simulink model "Scenario_3_v2"  (R2020b)
settings: Solver=ode1be  StartTime=0.0  StopTime=0.5  FixedStep=Ts  MaxStep=Ts/10  MinStep=Ts/40  RelTol=1e-3
values from neighbouring files (symbols this model uses):
  c0 = c0_zeb    (= 6.57988e-09)    [Scenario_17_parameters_v2.m]    (also in Scenario_1_parameters_v2.m; Scenario_2_parameters_v2.m; Scenario_3_parameters_v2.m)
  c0_hawk = 6.37282e-09    [Scenario_17_parameters_v2.m]    (also in Scenario_1_parameters_v2.m; Scenario_2_parameters_v2.m; Scenario_3_parameters_v2.m)
  c1 = c1_zeb    (= 9.15905e-09)    [Scenario_17_parameters_v2.m]    (also in Scenario_1_parameters_v2.m; Scenario_2_parameters_v2.m; Scenario_3_parameters_v2.m)
  c1_hawk = 8.76156e-09    [Scenario_17_parameters_v2.m]    (also in Scenario_1_parameters_v2.m; Scenario_2_parameters_v2.m; Scenario_3_parameters_v2.m)
  fg = 50    [Scenario_17_parameters_v2.m]    (also in Scenario_1_parameters_v2.m; Scenario_2_parameters_v2.m; Scenario_3_parameters_v2.m)
  G10gen = 0.90    (= 0.9)    [Scenario_3_parameters_v2.m]
  G12gen = 0.85    [Scenario_3_parameters_v2.m]
  G1gen = 0.4692    [Scenario_17_parameters_v2.m]    (also in Scenario_1_parameters_v2.m = 0.1; Scenario_2_parameters_v2.m = 0.298581; Scenario_3_parameters_v2.m = 0.65)
  G2gen = 0.80    (= 0.8)    [Scenario_1_parameters_v2.m]    (also in Scenario_2_parameters_v2.m = 0.7; Scenario_3_parameters_v2.m = 0.4)
  G3gen = 0.85    [Scenario_1_parameters_v2.m]    (also in Scenario_2_parameters_v2.m = 0.9; Scenario_3_parameters_v2.m = 0.6)
  G4gen = 0.65    [Scenario_3_parameters_v2.m]
  G5gen = 0.75    [Scenario_17_parameters_v2.m]    (also in Scenario_1_parameters_v2.m = 0.8; Scenario_2_parameters_v2.m = 0.8; Scenario_3_parameters_v2.m = 0.705)
  G6gen = 0.90    (= 0.9)    [Scenario_17_parameters_v2.m]    (also in Scenario_1_parameters_v2.m; Scenario_2_parameters_v2.m = 0.81797; Scenario_3_parameters_v2.m = 0.45)
  G7gen = 0.20    (= 0.2)    [Scenario_17_parameters_v2.m]    (also in Scenario_1_parameters_v2.m = 0.5227; Scenario_2_parameters_v2.m = 0.5098; Scenario_3_parameters_v2.m = 0.4)
  G8gen = 0.58    [Scenario_17_parameters_v2.m]    (also in Scenario_3_parameters_v2.m = 0.65)
  G9gen = 0.8833    [Scenario_17_parameters_v2.m]    (also in Scenario_3_parameters_v2.m = 0.9)
  Iovc = 1.2    [Scenario_17_parameters_v2.m]    (also in Scenario_1_parameters_v2.m; Scenario_2_parameters_v2.m; Scenario_3_parameters_v2.m)
  l0 = l0_zeb    (= 0.00368)    [Scenario_17_parameters_v2.m]    (also in Scenario_1_parameters_v2.m; Scenario_2_parameters_v2.m; Scenario_3_parameters_v2.m)
  l0_hawk = 0.00373    [Scenario_17_parameters_v2.m]    (also in Scenario_1_parameters_v2.m; Scenario_2_parameters_v2.m; Scenario_3_parameters_v2.m)
  l1 = l1_zeb    (= 0.00128)    [Scenario_17_parameters_v2.m]    (also in Scenario_1_parameters_v2.m; Scenario_2_parameters_v2.m; Scenario_3_parameters_v2.m)
  L10dem = 0.04    [Scenario_3_parameters_v2.m]
  L12dem = 0.01    [Scenario_17_parameters_v2.m]    (also in Scenario_3_parameters_v2.m = 0.02)
  L13dem = 0.01    [Scenario_3_parameters_v2.m]
  l1_hawk = 0.00133    [Scenario_17_parameters_v2.m]    (also in Scenario_1_parameters_v2.m; Scenario_2_parameters_v2.m; Scenario_3_parameters_v2.m)
  L1dem = 0.25    [Scenario_17_parameters_v2.m]    (also in Scenario_3_parameters_v2.m = 0.1)
  L3dem = 0.30    (= 0.3)    [Scenario_17_parameters_v2.m]    (also in Scenario_1_parameters_v2.m = 0.1; Scenario_2_parameters_v2.m = 0.1; Scenario_3_parameters_v2.m = 0.2)
  L5dem = 0.25    [Scenario_17_parameters_v2.m]    (also in Scenario_1_parameters_v2.m = 0.35; Scenario_2_parameters_v2.m = 0.35; Scenario_3_parameters_v2.m = 0.1)
  L6dem = 0.15    [Scenario_1_parameters_v2.m]    (also in Scenario_2_parameters_v2.m; Scenario_3_parameters_v2.m = 0.1)
  L7dem = 0.10    (= 0.1)    [Scenario_1_parameters_v2.m]    (also in Scenario_2_parameters_v2.m; Scenario_3_parameters_v2.m = 0.2)
  L9dem = 0.15    [Scenario_17_parameters_v2.m]    (also in Scenario_3_parameters_v2.m = 0.1)
  Pr = Sr*PF    (= 1600500000)    [Scenario_17_parameters_v2.m]    (also in Scenario_1_parameters_v2.m = 1472500000; Scenario_2_parameters_v2.m = 1805000000; Scenario_3_parameters_v2.m = 12740000000)
  Qr = sqrt(Sr^2 - Pr^2)    [Scenario_17_parameters_v2.m]    (also in Scenario_1_parameters_v2.m; Scenario_2_parameters_v2.m; Scenario_3_parameters_v2.m)
  r0 = r0_zeb    (= 0.39362)    [Scenario_17_parameters_v2.m]    (also in Scenario_1_parameters_v2.m; Scenario_2_parameters_v2.m; Scenario_3_parameters_v2.m)
  r0_hawk = 0.44587    [Scenario_17_parameters_v2.m]    (also in Scenario_1_parameters_v2.m; Scenario_2_parameters_v2.m; Scenario_3_parameters_v2.m)
  r1 = r1_zeb    (= 0.06862)    [Scenario_17_parameters_v2.m]    (also in Scenario_1_parameters_v2.m; Scenario_2_parameters_v2.m; Scenario_3_parameters_v2.m)
  r1_hawk = 0.12087    [Scenario_17_parameters_v2.m]    (also in Scenario_1_parameters_v2.m; Scenario_2_parameters_v2.m; Scenario_3_parameters_v2.m)
  Rtpu = Xtpu/40    (= 0.0025)    [Scenario_17_parameters_v2.m]    (also in Scenario_1_parameters_v2.m = 0.00375; Scenario_2_parameters_v2.m = 0.00375; Scenario_3_parameters_v2.m)
  S10non = 500e6    (= 500000000)    [Scenario_3_parameters_v2.m]
  S12non = 250e6    (= 250000000)    [Scenario_3_parameters_v2.m]
  S1non = 700e6    (= 700000000)    [Scenario_17_parameters_v2.m]    (also in Scenario_1_parameters_v2.m = 400000000; Scenario_2_parameters_v2.m = 400000000; Scenario_3_parameters_v2.m = 1000000000)
  S2non = 300e6    (= 300000000)    [Scenario_1_parameters_v2.m]    (also in Scenario_2_parameters_v2.m; Scenario_3_parameters_v2.m = 3000000000)
  S3non = 200e6    (= 200000000)    [Scenario_1_parameters_v2.m]    (also in Scenario_2_parameters_v2.m; Scenario_3_parameters_v2.m = 1000000000)
  S4non = 2000e6    (= 2000000000)    [Scenario_3_parameters_v2.m]
  S5non = 400e6    (= 400000000)    [Scenario_17_parameters_v2.m]    (also in Scenario_1_parameters_v2.m = 500000000; Scenario_2_parameters_v2.m = 500000000; Scenario_3_parameters_v2.m = 2000000000)
  S6non = 150e6    (= 150000000)    [Scenario_17_parameters_v2.m]    (also in Scenario_1_parameters_v2.m = 400000000; Scenario_2_parameters_v2.m = 400000000; Scenario_3_parameters_v2.m = 3000000000)
  S7non = 1500e6    (= 1500000000)    [Scenario_17_parameters_v2.m]    (also in Scenario_1_parameters_v2.m = 200000000; Scenario_2_parameters_v2.m = 200000000; Scenario_3_parameters_v2.m = 4000000000)
  S8non = 600e6    (= 600000000)    [Scenario_17_parameters_v2.m]    (also in Scenario_3_parameters_v2.m = 2000000000)
  S9non = 200e6    (= 200000000)    [Scenario_17_parameters_v2.m]    (also in Scenario_3_parameters_v2.m = 1500000000)
  tonvsc = 0    [Scenario_17_parameters_v2.m]    (also in Scenario_1_parameters_v2.m; Scenario_2_parameters_v2.m; Scenario_3_parameters_v2.m = 0.0001)
  Ts = 50e-6    (= 5e-05)    [Scenario_17_parameters_v2.m]    (also in Scenario_1_parameters_v2.m = 0.0002; Scenario_2_parameters_v2.m = 2e-05; Scenario_3_parameters_v2.m = 0.0001)
  Vhv = 220e3    (= 220000)    [Scenario_17_parameters_v2.m]    (also in Scenario_1_parameters_v2.m; Scenario_2_parameters_v2.m; Scenario_3_parameters_v2.m)
  Vmv = 22e3    (= 22000)    [Scenario_17_parameters_v2.m]    (also in Scenario_1_parameters_v2.m; Scenario_2_parameters_v2.m; Scenario_3_parameters_v2.m)
  w_pll = 2*pi*80    (= 502.654824574)    [Scenario_17_parameters_v2.m]    (also in Scenario_1_parameters_v2.m; Scenario_2_parameters_v2.m; Scenario_3_parameters_v2.m)
  wc1 = wsw1/10    (= 848.230016469)    [Scenario_17_parameters_v2.m]    (also in Scenario_1_parameters_v2.m; Scenario_2_parameters_v2.m; Scenario_3_parameters_v2.m)
  wdc1 = wc1/10    (= 84.8230016469)    [Scenario_17_parameters_v2.m]    (also in Scenario_1_parameters_v2.m; Scenario_2_parameters_v2.m; Scenario_3_parameters_v2.m)
  wpq1 = wc1/10    (= 84.8230016469)    [Scenario_17_parameters_v2.m]    (also in Scenario_1_parameters_v2.m; Scenario_2_parameters_v2.m; Scenario_3_parameters_v2.m)
  wsw1 = ksw1*2*pi*fg    (= 8482.30016469)    [Scenario_17_parameters_v2.m]    (also in Scenario_1_parameters_v2.m; Scenario_2_parameters_v2.m; Scenario_3_parameters_v2.m)
  Xtpu = 0.10    (= 0.1)    [Scenario_17_parameters_v2.m]    (also in Scenario_1_parameters_v2.m = 0.15; Scenario_2_parameters_v2.m = 0.15; Scenario_3_parameters_v2.m)
undefined symbols (not defined in the file or in its folder): D11, Delta
libraries: powerlib x428, simulink_extras x272, powerlib_meascontrol x194, pid_lib x105, simulink x60, eeTransforms x54, spsFirstOrderFilterLib x36, eePwmGeneratorTwoLevel x9
(part 39 of 40)

== system Scenario_3_v2/G4/VSC v2/VSC Control/Control loops/Phasor PQ 1st/Outer-loop/Power calculation ==
  note: AC power calculation using symmetrical components in dq axis
  note: Pavgp = 3/2*(vqp*iqp + vdp*idp) and Qavgp = 3/2*(vqp*idp-vdp*iqp)
  note: P = Pavg + Pc2*cos(2wt) + Ps2*sin(2wt) ---> Pavg = Pavgp + Pavgn
  note: Q = Qavg + Qc2*cos(2wt) + Qs2*sin(2wt) ---> Qavg = Qavgp + Qavgn
  note: Pavgn = 3/2*(vqn*iqn + vdn*idn) and Qavgn = 3/2*(vqn*idn-vdn*iqn)
  vq+ : Inport
  vd+ : Inport  Port=2
  iq+ : Inport  Port=3
  id+ : Inport  Port=4
  vq- : Inport  Port=5
  vd- : Inport  Port=6
  iq- : Inport  Port=7
  id- : Inport  Port=8
  Gain : Gain  Gain=3/2
  Gain1 : Gain  Gain=3/2
  Gain2 : Gain  Gain=-1
  Gain3 : Gain  Gain=-1
  Gain4 : Gain  Gain=negseq_en
  Mux{,1..3} (4 alike) : Mux  Inputs=2
  Product{,1..3} (4 alike) : Product
  Sum1 : Sum
  Sum2 : Sum
  Sum8 : Sum
  PQ : Outport
  wires:
  Sum8/1 -> Gain/1
  Gain2/1 -> Mux2/2
  Mux2/1 -> Product2/2
  Product2/1 -> Sum8/2
  Mux/1 -> Product/2
  Product/1 -> Sum8/1
  iq+/1 -> [iqp]
  [iqp] -> Gain2/1, Mux/1
  id+/1 -> [idp]
  [idp] -> Mux2/1, Mux/2
  vq+/1 -> [vqp]
  [vqp] -> Product/1
  vd+/1 -> [vdp]
  [vdp] -> Product2/1
  Gain/1 -> Sum1/1
  Sum1/1 -> PQ/1
  Gain3/1 -> Mux3/2
  Mux1/1 -> Product1/2
  Product3/1 -> Sum2/2
  Product1/1 -> Sum2/1
  [vdn] -> Product3/1
  Mux3/1 -> Product3/2
  [vqn] -> Product1/1
  Sum2/1 -> Gain1/1
  [iqn] -> Gain3/1, Mux1/1
  [idn] -> Mux3/1, Mux1/2
  vq-/1 -> [vqn]
  vd-/1 -> [vdn]
  iq-/1 -> [iqn]
  id-/1 -> [idn]
  Gain1/1 -> Gain4/1
  Gain4/1 -> Sum1/2

== system Scenario_3_v2/G4/VSC v2/VSC Control/Control loops/SW, EMT AVG, Phasor Quasi-EMT/Outer-loop/Power calculation ==
  note: AC power calculation using symmetrical components in dq axis
  note: Pavgp = 3/2*(vqp*iqp + vdp*idp) and Qavgp = 3/2*(vqp*idp-vdp*iqp)
  note: P = Pavg + Pc2*cos(2wt) + Ps2*sin(2wt) ---> Pavg = Pavgp + Pavgn
  note: Q = Qavg + Qc2*cos(2wt) + Qs2*sin(2wt) ---> Qavg = Qavgp + Qavgn
  note: Pavgn = 3/2*(vqn*iqn + vdn*idn) and Qavgn = 3/2*(vqn*idn-vdn*iqn)
  vq+ : Inport
  vd+ : Inport  Port=2
  iq+ : Inport  Port=3
  id+ : Inport  Port=4
  vq- : Inport  Port=5
  vd- : Inport  Port=6
  iq- : Inport  Port=7
  id- : Inport  Port=8
  Gain : Gain  Gain=3/2
  Gain1 : Gain  Gain=3/2
  Gain2 : Gain  Gain=-1
  Gain3 : Gain  Gain=-1
  Gain4 : Gain  Gain=negseq_en
  Mux{,1..3} (4 alike) : Mux  Inputs=2
  Product{,1..3} (4 alike) : Product
  Sum1 : Sum
  Sum2 : Sum
  Sum8 : Sum
  PQ : Outport
  wires:
  Sum8/1 -> Gain/1
  Gain2/1 -> Mux2/2
  Mux2/1 -> Product2/2
  Product2/1 -> Sum8/2
  Mux/1 -> Product/2
  Product/1 -> Sum8/1
  iq+/1 -> [iqp]
  [iqp] -> Gain2/1, Mux/1
  id+/1 -> [idp]
  [idp] -> Mux2/1, Mux/2
  vq+/1 -> [vqp]
  [vqp] -> Product/1
  vd+/1 -> [vdp]
  [vdp] -> Product2/1
  Gain/1 -> Sum1/1
  Sum1/1 -> PQ/1
  Gain3/1 -> Mux3/2
  Mux1/1 -> Product1/2
  Product3/1 -> Sum2/2
  Product1/1 -> Sum2/1
  [vdn] -> Product3/1
  Mux3/1 -> Product3/2
  [vqn] -> Product1/1
  Sum2/1 -> Gain1/1
  [iqn] -> Gain3/1, Mux1/1
  [idn] -> Mux3/1, Mux1/2
  vq-/1 -> [vqn]
  vd-/1 -> [vdn]
  iq-/1 -> [iqn]
  id-/1 -> [idn]
  Gain1/1 -> Gain4/1
  Gain4/1 -> Sum1/2

== system Scenario_3_v2/G4/VSC v2/VSC Control/Control loops/SW, EMT AVG, Phasor Quasi-EMT/Outer-loop/Subsystem2 ==
  note: Hold initial variable value for a given time
  In1 : Inport
  Constant : Constant  Value=x0
  Constant1 : Constant
  Integrator : Integrator
  Switch : Switch  Threshold=Td
  Out1 : Outport
  wires:
  Integrator/1 -> Switch/2
  In1/1 -> Switch/1
  Switch/1 -> Out1/1
  Constant/1 -> Switch/3
  Constant1/1 -> Integrator/1

== system Scenario_3_v2/G4/VSC v2/VSC Control/Control loops/SW, EMT AVG, Phasor Quasi-EMT/Outer-loop/Subsystem3 ==
  note: Hold initial variable value for a given time
  In1 : Inport
  Constant : Constant  Value=x0
  Constant1 : Constant
  Integrator : Integrator
  Switch : Switch  Threshold=Td
  Out1 : Outport
  wires:
  Integrator/1 -> Switch/2
  In1/1 -> Switch/1
  Switch/1 -> Out1/1
  Constant/1 -> Switch/3
  Constant1/1 -> Integrator/1

== system Scenario_3_v2/G4/VSC v2/VSC Control/Measurements/EMT/PLL aligned with positive-sequence/Phase-sequence separation ==
  note: Phase-sequence separation based on
      | Delayed Signal Cancellation (DSC) method
  abc : Inport
  Theta : Inport  Port=2
  Complex to Real-Imag1 : ComplexToRealImag
  Complex to Real-Imag2 : ComplexToRealImag
  Complex to Real-Imag3 : ComplexToRealImag
  Constant : Constant  Value=negseq_en
  Demux3 : Demux  Outputs=3
  Exp2 : Math  OutputSignalType=complex  SaturateOnIntegerOverflow=on
  Exp3 : Math  OutputSignalType=complex  SaturateOnIntegerOverflow=on
  Gain1 : Gain  Gain=1/2
  Gain4 : Gain  Gain=-1i
  Gain5 : Gain  Gain=1i
  Gain6 : Gain  Gain=1/2
  Gain7 : Gain  Gain=1i
  NOT : Logic  Operator=NOT  IconShape=distinctive  AllPortsSameDT=off  OutDataTypeStr=boolean
  Product3 : Product
  Product4 : Product
  Real-Imag to Complex : RealImagToComplex
  Real-Imag to Complex1 : RealImagToComplex
  Sum1 : Sum  Inputs=|++
  Sum2 : Sum  Inputs=-+|
  Switch : Switch  Criteria=u2 ~= 0
  Terminator3 : Terminator
  Transport Delay2 : TransportDelay  DelayTime=1/4*(1/fg)  BufferSize=1024*4
  Transport Delay3 : TransportDelay  DelayTime=1/4*(1/fg)  BufferSize=1024*4
  abc to Alpha-Beta-Zero : powerlib_meascontrol/Transformations/abc to Alpha-Beta-Zero
  q+ : Outport
  d+ : Outport  Port=2
  q- : Outport  Port=3
  d- : Outport  Port=4
  wires:
  NOT/1 -> Switch/2
  Constant/1 -> NOT/1
  Switch/1 -> Product3/1
  Gain6/1 -> Switch/3
  Sum2/1 -> Gain1/1
  Transport Delay2/1 -> Real-Imag to Complex1/1
  Demux3/1 -> Real-Imag to Complex/1
  Complex to Real-Imag1/2 -> Transport Delay3/1
  Gain1/1 -> Product4/2
  Real-Imag to Complex/1 -> Complex to Real-Imag1/1, Sum2/2, Sum1/1, Switch/1
  Complex to Real-Imag3/1 -> d-/1
  Real-Imag to Complex1/1 -> Gain5/1
  Complex to Real-Imag1/1 -> Transport Delay2/1
  Transport Delay3/1 -> Real-Imag to Complex1/2
  Demux3/2 -> Real-Imag to Complex/2
  Product3/1 -> Complex to Real-Imag2/1
  Product4/1 -> Complex to Real-Imag3/1
  abc to Alpha-Beta-Zero/1 -> Demux3/1
  abc/1 -> abc to Alpha-Beta-Zero/1
  Exp3/1 -> Product4/1
  Complex to Real-Imag3/2 -> q-/1
  Complex to Real-Imag2/2 -> q+/1
  Demux3/3 -> Terminator3/1
  Sum1/1 -> Gain6/1
  Gain5/1 -> Sum2/1, Sum1/2
  Exp2/1 -> Product3/2
  Gain4/1 -> Exp2/1
  Theta/1 -> Gain4/1, Gain7/1
  Gain7/1 -> Exp3/1
  Complex to Real-Imag2/1 -> d+/1

== system Scenario_3_v2/G4/VSC v2/VSC Control/Measurements/EMT/PLL aligned with positive-sequence/Subsystem ==
  note: PI controller with reset port and initial conditions restored after reset or after maximum/minimum values are reached
  in : Inport
  Reset : Inport  Port=2
  Compare To Constant2 : simulink/Logic and Bit Operations/Compare To Constant  relop=~=  const=0  OutDataTypeStr=boolean
  Constant2 : Constant  Value=2*pi*fg
  Gain : Gain  Gain=kp_pll
  Gain1 : Gain  Gain=kp_pll/tau_pll
  Integrator Limited : Integrator  ExternalReset=level  InitialCondition=2*pi*fg  UpperSaturationLimit=10.1*2*pi*fg  LowerSaturationLimit=0.09*2*pi*fg  ShowSaturationPort=on
  Memory1 : Memory
  NOT : Logic  Operator=NOT  IconShape=distinctive  AllPortsSameDT=off  OutDataTypeStr=boolean
  OR2 : Logic  Operator=OR  IconShape=distinctive  AllPortsSameDT=off  OutDataTypeStr=boolean
  Product : Product
  Sum : Sum
  Switch1 : Switch
  w : Outport
  wires:
  Switch1/1 -> w/1
  Product/1 -> Gain1/1, Gain/1
  Gain1/1 -> Integrator Limited/1
  Integrator Limited/2 -> Compare To Constant2/1, Switch1/2
  Compare To Constant2/1 -> Memory1/1
  OR2/1 -> Integrator Limited/2, NOT/1
  Constant2/1 -> Switch1/3
  Memory1/1 -> OR2/1
  Reset/1 -> OR2/2
  Gain/1 -> Sum/1
  Integrator Limited/1 -> Sum/2
  Sum/1 -> Switch1/1
  in/1 -> Product/1
  NOT/1 -> Product/2

== system Scenario_3_v2/G6/VSC v2/VSC Control/Control loops/Phasor I 1st/Outer-loop/Power calculation ==
  note: AC power calculation using symmetrical components in dq axis
  note: Pavgp = 3/2*(vqp*iqp + vdp*idp) and Qavgp = 3/2*(vqp*idp-vdp*iqp)
  note: P = Pavg + Pc2*cos(2wt) + Ps2*sin(2wt) ---> Pavg = Pavgp + Pavgn
  note: Q = Qavg + Qc2*cos(2wt) + Qs2*sin(2wt) ---> Qavg = Qavgp + Qavgn
  note: Pavgn = 3/2*(vqn*iqn + vdn*idn) and Qavgn = 3/2*(vqn*idn-vdn*iqn)
  vq+ : Inport
  vd+ : Inport  Port=2
  iq+ : Inport  Port=3
  id+ : Inport  Port=4
  vq- : Inport  Port=5
  vd- : Inport  Port=6
  iq- : Inport  Port=7
  id- : Inport  Port=8
  Gain : Gain  Gain=3/2
  Gain1 : Gain  Gain=3/2
  Gain2 : Gain  Gain=-1
  Gain3 : Gain  Gain=-1
  Gain4 : Gain  Gain=negseq_en
  Mux{,1..3} (4 alike) : Mux  Inputs=2
  Product{,1..3} (4 alike) : Product
  Sum1 : Sum
  Sum2 : Sum
  Sum8 : Sum
  PQ : Outport
  wires:
  Sum8/1 -> Gain/1
  Gain2/1 -> Mux2/2
  Mux2/1 -> Product2/2
  Product2/1 -> Sum8/2
  Mux/1 -> Product/2
  Product/1 -> Sum8/1
  iq+/1 -> [iqp]
  [iqp] -> Gain2/1, Mux/1
  id+/1 -> [idp]
  [idp] -> Mux2/1, Mux/2
  vq+/1 -> [vqp]
  [vqp] -> Product/1
  vd+/1 -> [vdp]
  [vdp] -> Product2/1
  Gain/1 -> Sum1/1
  Sum1/1 -> PQ/1
  Gain3/1 -> Mux3/2
  Mux1/1 -> Product1/2
  Product3/1 -> Sum2/2
  Product1/1 -> Sum2/1
  [vdn] -> Product3/1
  Mux3/1 -> Product3/2
  [vqn] -> Product1/1
  Sum2/1 -> Gain1/1
  [iqn] -> Gain3/1, Mux1/1
  [idn] -> Mux3/1, Mux1/2
  vq-/1 -> [vqn]
  vd-/1 -> [vdn]
  iq-/1 -> [iqn]
  id-/1 -> [idn]
  Gain1/1 -> Gain4/1
  Gain4/1 -> Sum1/2

== system Scenario_3_v2/G6/VSC v2/VSC Control/Control loops/Phasor I ref/Outer-loop/Power calculation ==
  note: AC power calculation using symmetrical components in dq axis
  note: Pavgp = 3/2*(vqp*iqp + vdp*idp) and Qavgp = 3/2*(vqp*idp-vdp*iqp)
  note: P = Pavg + Pc2*cos(2wt) + Ps2*sin(2wt) ---> Pavg = Pavgp + Pavgn
  note: Q = Qavg + Qc2*cos(2wt) + Qs2*sin(2wt) ---> Qavg = Qavgp + Qavgn
  note: Pavgn = 3/2*(vqn*iqn + vdn*idn) and Qavgn = 3/2*(vqn*idn-vdn*iqn)
  vq+ : Inport
  vd+ : Inport  Port=2
  iq+ : Inport  Port=3
  id+ : Inport  Port=4
  vq- : Inport  Port=5
  vd- : Inport  Port=6
  iq- : Inport  Port=7
  id- : Inport  Port=8
  Gain : Gain  Gain=3/2
  Gain1 : Gain  Gain=3/2
  Gain2 : Gain  Gain=-1
  Gain3 : Gain  Gain=-1
  Gain4 : Gain  Gain=negseq_en
  Mux{,1..3} (4 alike) : Mux  Inputs=2
  Product{,1..3} (4 alike) : Product
  Sum1 : Sum
  Sum2 : Sum
  Sum8 : Sum
  PQ : Outport
  wires:
  Sum8/1 -> Gain/1
  Gain2/1 -> Mux2/2
  Mux2/1 -> Product2/2
  Product2/1 -> Sum8/2
  Mux/1 -> Product/2
  Product/1 -> Sum8/1
  iq+/1 -> [iqp]
  [iqp] -> Gain2/1, Mux/1
  id+/1 -> [idp]
  [idp] -> Mux2/1, Mux/2
  vq+/1 -> [vqp]
  [vqp] -> Product/1
  vd+/1 -> [vdp]
  [vdp] -> Product2/1
  Gain/1 -> Sum1/1
  Sum1/1 -> PQ/1
  Gain3/1 -> Mux3/2
  Mux1/1 -> Product1/2
  Product3/1 -> Sum2/2
  Product1/1 -> Sum2/1
  [vdn] -> Product3/1
  Mux3/1 -> Product3/2
  [vqn] -> Product1/1
  Sum2/1 -> Gain1/1
  [iqn] -> Gain3/1, Mux1/1
  [idn] -> Mux3/1, Mux1/2
  vq-/1 -> [vqn]
  vd-/1 -> [vdn]
  iq-/1 -> [iqn]
  id-/1 -> [idn]
  Gain1/1 -> Gain4/1
  Gain4/1 -> Sum1/2

== system Scenario_3_v2/G6/VSC v2/VSC Control/Control loops/Phasor PQ 1st/Outer-loop/Power calculation ==
  note: AC power calculation using symmetrical components in dq axis
  note: Pavgp = 3/2*(vqp*iqp + vdp*idp) and Qavgp = 3/2*(vqp*idp-vdp*iqp)
  note: P = Pavg + Pc2*cos(2wt) + Ps2*sin(2wt) ---> Pavg = Pavgp + Pavgn
  note: Q = Qavg + Qc2*cos(2wt) + Qs2*sin(2wt) ---> Qavg = Qavgp + Qavgn
  note: Pavgn = 3/2*(vqn*iqn + vdn*idn) and Qavgn = 3/2*(vqn*idn-vdn*iqn)
  vq+ : Inport
  vd+ : Inport  Port=2
  iq+ : Inport  Port=3
  id+ : Inport  Port=4
  vq- : Inport  Port=5
  vd- : Inport  Port=6
  iq- : Inport  Port=7
  id- : Inport  Port=8
  Gain : Gain  Gain=3/2
  Gain1 : Gain  Gain=3/2
  Gain2 : Gain  Gain=-1
  Gain3 : Gain  Gain=-1
  Gain4 : Gain  Gain=negseq_en
  Mux{,1..3} (4 alike) : Mux  Inputs=2
  Product{,1..3} (4 alike) : Product
  Sum1 : Sum
  Sum2 : Sum
  Sum8 : Sum
  PQ : Outport
  wires:
  Sum8/1 -> Gain/1
  Gain2/1 -> Mux2/2
  Mux2/1 -> Product2/2
  Product2/1 -> Sum8/2
  Mux/1 -> Product/2
  Product/1 -> Sum8/1
  iq+/1 -> [iqp]
  [iqp] -> Gain2/1, Mux/1
  id+/1 -> [idp]
  [idp] -> Mux2/1, Mux/2
  vq+/1 -> [vqp]
  [vqp] -> Product/1
  vd+/1 -> [vdp]
  [vdp] -> Product2/1
  Gain/1 -> Sum1/1
  Sum1/1 -> PQ/1
  Gain3/1 -> Mux3/2
  Mux1/1 -> Product1/2
  Product3/1 -> Sum2/2
  Product1/1 -> Sum2/1
  [vdn] -> Product3/1
  Mux3/1 -> Product3/2
  [vqn] -> Product1/1
  Sum2/1 -> Gain1/1
  [iqn] -> Gain3/1, Mux1/1
  [idn] -> Mux3/1, Mux1/2
  vq-/1 -> [vqn]
  vd-/1 -> [vdn]
  iq-/1 -> [iqn]
  id-/1 -> [idn]
  Gain1/1 -> Gain4/1
  Gain4/1 -> Sum1/2

== system Scenario_3_v2/G6/VSC v2/VSC Control/Control loops/SW, EMT AVG, Phasor Quasi-EMT/Outer-loop/Power calculation ==
  note: AC power calculation using symmetrical components in dq axis
  note: Pavgp = 3/2*(vqp*iqp + vdp*idp) and Qavgp = 3/2*(vqp*idp-vdp*iqp)
  note: P = Pavg + Pc2*cos(2wt) + Ps2*sin(2wt) ---> Pavg = Pavgp + Pavgn
  note: Q = Qavg + Qc2*cos(2wt) + Qs2*sin(2wt) ---> Qavg = Qavgp + Qavgn
  note: Pavgn = 3/2*(vqn*iqn + vdn*idn) and Qavgn = 3/2*(vqn*idn-vdn*iqn)
  vq+ : Inport
  vd+ : Inport  Port=2
  iq+ : Inport  Port=3
  id+ : Inport  Port=4
  vq- : Inport  Port=5
  vd- : Inport  Port=6
  iq- : Inport  Port=7
  id- : Inport  Port=8
  Gain : Gain  Gain=3/2
  Gain1 : Gain  Gain=3/2
  Gain2 : Gain  Gain=-1
  Gain3 : Gain  Gain=-1
  Gain4 : Gain  Gain=negseq_en
  Mux{,1..3} (4 alike) : Mux  Inputs=2
  Product{,1..3} (4 alike) : Product
  Sum1 : Sum
  Sum2 : Sum
  Sum8 : Sum
  PQ : Outport
  wires:
  Sum8/1 -> Gain/1
  Gain2/1 -> Mux2/2
  Mux2/1 -> Product2/2
  Product2/1 -> Sum8/2
  Mux/1 -> Product/2
  Product/1 -> Sum8/1
  iq+/1 -> [iqp]
  [iqp] -> Gain2/1, Mux/1
  id+/1 -> [idp]
  [idp] -> Mux2/1, Mux/2
  vq+/1 -> [vqp]
  [vqp] -> Product/1
  vd+/1 -> [vdp]
  [vdp] -> Product2/1
  Gain/1 -> Sum1/1
  Sum1/1 -> PQ/1
  Gain3/1 -> Mux3/2
  Mux1/1 -> Product1/2
  Product3/1 -> Sum2/2
  Product1/1 -> Sum2/1
  [vdn] -> Product3/1
  Mux3/1 -> Product3/2
  [vqn] -> Product1/1
  Sum2/1 -> Gain1/1
  [iqn] -> Gain3/1, Mux1/1
  [idn] -> Mux3/1, Mux1/2
  vq-/1 -> [vqn]
  vd-/1 -> [vdn]
  iq-/1 -> [iqn]
  id-/1 -> [idn]
  Gain1/1 -> Gain4/1
  Gain4/1 -> Sum1/2

== system Scenario_3_v2/G6/VSC v2/VSC Control/Control loops/SW, EMT AVG, Phasor Quasi-EMT/Outer-loop/Subsystem2 ==
  note: Hold initial variable value for a given time
  In1 : Inport
  Constant : Constant  Value=x0
  Constant1 : Constant
  Integrator : Integrator
  Switch : Switch  Threshold=Td
  Out1 : Outport
  wires:
  Integrator/1 -> Switch/2
  In1/1 -> Switch/1
  Switch/1 -> Out1/1
  Constant/1 -> Switch/3
  Constant1/1 -> Integrator/1

== system Scenario_3_v2/G6/VSC v2/VSC Control/Control loops/SW, EMT AVG, Phasor Quasi-EMT/Outer-loop/Subsystem3 ==
  note: Hold initial variable value for a given time
  In1 : Inport
  Constant : Constant  Value=x0
  Constant1 : Constant
  Integrator : Integrator
  Switch : Switch  Threshold=Td
  Out1 : Outport
  wires:
  Integrator/1 -> Switch/2
  In1/1 -> Switch/1
  Switch/1 -> Out1/1
  Constant/1 -> Switch/3
  Constant1/1 -> Integrator/1

== system Scenario_3_v2/G6/VSC v2/VSC Control/Measurements/EMT/PLL aligned with positive-sequence/Phase-sequence separation ==
  note: Phase-sequence separation based on
      | Delayed Signal Cancellation (DSC) method
  abc : Inport
  Theta : Inport  Port=2
  Complex to Real-Imag1 : ComplexToRealImag
  Complex to Real-Imag2 : ComplexToRealImag
  Complex to Real-Imag3 : ComplexToRealImag
  Constant : Constant  Value=negseq_en
  Demux3 : Demux  Outputs=3
  Exp2 : Math  OutputSignalType=complex  SaturateOnIntegerOverflow=on
  Exp3 : Math  OutputSignalType=complex  SaturateOnIntegerOverflow=on
  Gain1 : Gain  Gain=1/2
  Gain4 : Gain  Gain=-1i
  Gain5 : Gain  Gain=1i
  Gain6 : Gain  Gain=1/2
  Gain7 : Gain  Gain=1i
  NOT : Logic  Operator=NOT  IconShape=distinctive  AllPortsSameDT=off  OutDataTypeStr=boolean
  Product3 : Product
  Product4 : Product
  Real-Imag to Complex : RealImagToComplex
  Real-Imag to Complex1 : RealImagToComplex
  Sum1 : Sum  Inputs=|++
  Sum2 : Sum  Inputs=-+|
  Switch : Switch  Criteria=u2 ~= 0
  Terminator3 : Terminator
  Transport Delay2 : TransportDelay  DelayTime=1/4*(1/fg)  BufferSize=1024*4
  Transport Delay3 : TransportDelay  DelayTime=1/4*(1/fg)  BufferSize=1024*4
  abc to Alpha-Beta-Zero : powerlib_meascontrol/Transformations/abc to Alpha-Beta-Zero
  q+ : Outport
  d+ : Outport  Port=2
  q- : Outport  Port=3
  d- : Outport  Port=4
  wires:
  NOT/1 -> Switch/2
  Constant/1 -> NOT/1
  Switch/1 -> Product3/1
  Gain6/1 -> Switch/3
  Sum2/1 -> Gain1/1
  Transport Delay2/1 -> Real-Imag to Complex1/1
  Demux3/1 -> Real-Imag to Complex/1
  Complex to Real-Imag1/2 -> Transport Delay3/1
  Gain1/1 -> Product4/2
  Real-Imag to Complex/1 -> Complex to Real-Imag1/1, Sum2/2, Sum1/1, Switch/1
  Complex to Real-Imag3/1 -> d-/1
  Real-Imag to Complex1/1 -> Gain5/1
  Complex to Real-Imag1/1 -> Transport Delay2/1
  Transport Delay3/1 -> Real-Imag to Complex1/2
  Demux3/2 -> Real-Imag to Complex/2
  Product3/1 -> Complex to Real-Imag2/1
  Product4/1 -> Complex to Real-Imag3/1
  abc to Alpha-Beta-Zero/1 -> Demux3/1
  abc/1 -> abc to Alpha-Beta-Zero/1
  Exp3/1 -> Product4/1
  Complex to Real-Imag3/2 -> q-/1
  Complex to Real-Imag2/2 -> q+/1
  Demux3/3 -> Terminator3/1
  Sum1/1 -> Gain6/1
  Gain5/1 -> Sum2/1, Sum1/2
  Exp2/1 -> Product3/2
  Gain4/1 -> Exp2/1
  Theta/1 -> Gain4/1, Gain7/1
  Gain7/1 -> Exp3/1
  Complex to Real-Imag2/1 -> d+/1

== system Scenario_3_v2/G6/VSC v2/VSC Control/Measurements/EMT/PLL aligned with positive-sequence/Subsystem ==
  note: PI controller with reset port and initial conditions restored after reset or after maximum/minimum values are reached
  in : Inport
  Reset : Inport  Port=2
  Compare To Constant2 : simulink/Logic and Bit Operations/Compare To Constant  relop=~=  const=0  OutDataTypeStr=boolean
  Constant2 : Constant  Value=2*pi*fg
  Gain : Gain  Gain=kp_pll
  Gain1 : Gain  Gain=kp_pll/tau_pll
  Integrator Limited : Integrator  ExternalReset=level  InitialCondition=2*pi*fg  UpperSaturationLimit=10.1*2*pi*fg  LowerSaturationLimit=0.09*2*pi*fg  ShowSaturationPort=on
  Memory1 : Memory
  NOT : Logic  Operator=NOT  IconShape=distinctive  AllPortsSameDT=off  OutDataTypeStr=boolean
  OR2 : Logic  Operator=OR  IconShape=distinctive  AllPortsSameDT=off  OutDataTypeStr=boolean
  Product : Product
  Sum : Sum
  Switch1 : Switch
  w : Outport
  wires:
  Switch1/1 -> w/1
  Product/1 -> Gain1/1, Gain/1
  Gain1/1 -> Integrator Limited/1
  Integrator Limited/2 -> Compare To Constant2/1, Switch1/2
  Compare To Constant2/1 -> Memory1/1
  OR2/1 -> Integrator Limited/2, NOT/1
  Constant2/1 -> Switch1/3
  Memory1/1 -> OR2/1
  Reset/1 -> OR2/2
  Gain/1 -> Sum/1
  Integrator Limited/1 -> Sum/2
  Sum/1 -> Switch1/1
  in/1 -> Product/1
  NOT/1 -> Product/2

== system Scenario_3_v2/G7/VSC v2/VSC Control/Control loops/Phasor I 1st/Outer-loop/Power calculation ==
  note: AC power calculation using symmetrical components in dq axis
  note: Pavgp = 3/2*(vqp*iqp + vdp*idp) and Qavgp = 3/2*(vqp*idp-vdp*iqp)
  note: P = Pavg + Pc2*cos(2wt) + Ps2*sin(2wt) ---> Pavg = Pavgp + Pavgn
  note: Q = Qavg + Qc2*cos(2wt) + Qs2*sin(2wt) ---> Qavg = Qavgp + Qavgn
  note: Pavgn = 3/2*(vqn*iqn + vdn*idn) and Qavgn = 3/2*(vqn*idn-vdn*iqn)
  vq+ : Inport
  vd+ : Inport  Port=2
  iq+ : Inport  Port=3
  id+ : Inport  Port=4
  vq- : Inport  Port=5
  vd- : Inport  Port=6
  iq- : Inport  Port=7
  id- : Inport  Port=8
  Gain : Gain  Gain=3/2
  Gain1 : Gain  Gain=3/2
  Gain2 : Gain  Gain=-1
  Gain3 : Gain  Gain=-1
  Gain4 : Gain  Gain=negseq_en
  Mux{,1..3} (4 alike) : Mux  Inputs=2
  Product{,1..3} (4 alike) : Product
  Sum1 : Sum
  Sum2 : Sum
  Sum8 : Sum
  PQ : Outport
  wires:
  Sum8/1 -> Gain/1
  Gain2/1 -> Mux2/2
  Mux2/1 -> Product2/2
  Product2/1 -> Sum8/2
  Mux/1 -> Product/2
  Product/1 -> Sum8/1
  iq+/1 -> [iqp]
  [iqp] -> Gain2/1, Mux/1
  id+/1 -> [idp]
  [idp] -> Mux2/1, Mux/2
  vq+/1 -> [vqp]
  [vqp] -> Product/1
  vd+/1 -> [vdp]
  [vdp] -> Product2/1
  Gain/1 -> Sum1/1
  Sum1/1 -> PQ/1
  Gain3/1 -> Mux3/2
  Mux1/1 -> Product1/2
  Product3/1 -> Sum2/2
  Product1/1 -> Sum2/1
  [vdn] -> Product3/1
  Mux3/1 -> Product3/2
  [vqn] -> Product1/1
  Sum2/1 -> Gain1/1
  [iqn] -> Gain3/1, Mux1/1
  [idn] -> Mux3/1, Mux1/2
  vq-/1 -> [vqn]
  vd-/1 -> [vdn]
  iq-/1 -> [iqn]
  id-/1 -> [idn]
  Gain1/1 -> Gain4/1
  Gain4/1 -> Sum1/2

== system Scenario_3_v2/G7/VSC v2/VSC Control/Control loops/Phasor I ref/Outer-loop/Power calculation ==
  note: AC power calculation using symmetrical components in dq axis
  note: Pavgp = 3/2*(vqp*iqp + vdp*idp) and Qavgp = 3/2*(vqp*idp-vdp*iqp)
  note: P = Pavg + Pc2*cos(2wt) + Ps2*sin(2wt) ---> Pavg = Pavgp + Pavgn
  note: Q = Qavg + Qc2*cos(2wt) + Qs2*sin(2wt) ---> Qavg = Qavgp + Qavgn
  note: Pavgn = 3/2*(vqn*iqn + vdn*idn) and Qavgn = 3/2*(vqn*idn-vdn*iqn)
  vq+ : Inport
  vd+ : Inport  Port=2
  iq+ : Inport  Port=3
  id+ : Inport  Port=4
  vq- : Inport  Port=5
  vd- : Inport  Port=6
  iq- : Inport  Port=7
  id- : Inport  Port=8
  Gain : Gain  Gain=3/2
  Gain1 : Gain  Gain=3/2
  Gain2 : Gain  Gain=-1
  Gain3 : Gain  Gain=-1
  Gain4 : Gain  Gain=negseq_en
  Mux{,1..3} (4 alike) : Mux  Inputs=2
  Product{,1..3} (4 alike) : Product
  Sum1 : Sum
  Sum2 : Sum
  Sum8 : Sum
  PQ : Outport
  wires:
  Sum8/1 -> Gain/1
  Gain2/1 -> Mux2/2
  Mux2/1 -> Product2/2
  Product2/1 -> Sum8/2
  Mux/1 -> Product/2
  Product/1 -> Sum8/1
  iq+/1 -> [iqp]
  [iqp] -> Gain2/1, Mux/1
  id+/1 -> [idp]
  [idp] -> Mux2/1, Mux/2
  vq+/1 -> [vqp]
  [vqp] -> Product/1
  vd+/1 -> [vdp]
  [vdp] -> Product2/1
  Gain/1 -> Sum1/1
  Sum1/1 -> PQ/1
  Gain3/1 -> Mux3/2
  Mux1/1 -> Product1/2
  Product3/1 -> Sum2/2
  Product1/1 -> Sum2/1
  [vdn] -> Product3/1
  Mux3/1 -> Product3/2
  [vqn] -> Product1/1
  Sum2/1 -> Gain1/1
  [iqn] -> Gain3/1, Mux1/1
  [idn] -> Mux3/1, Mux1/2
  vq-/1 -> [vqn]
  vd-/1 -> [vdn]
  iq-/1 -> [iqn]
  id-/1 -> [idn]
  Gain1/1 -> Gain4/1
  Gain4/1 -> Sum1/2

== system Scenario_3_v2/G7/VSC v2/VSC Control/Control loops/Phasor PQ 1st/Outer-loop/Power calculation ==
  note: AC power calculation using symmetrical components in dq axis
  note: Pavgp = 3/2*(vqp*iqp + vdp*idp) and Qavgp = 3/2*(vqp*idp-vdp*iqp)
  note: P = Pavg + Pc2*cos(2wt) + Ps2*sin(2wt) ---> Pavg = Pavgp + Pavgn
  note: Q = Qavg + Qc2*cos(2wt) + Qs2*sin(2wt) ---> Qavg = Qavgp + Qavgn
  note: Pavgn = 3/2*(vqn*iqn + vdn*idn) and Qavgn = 3/2*(vqn*idn-vdn*iqn)
  vq+ : Inport
  vd+ : Inport  Port=2
  iq+ : Inport  Port=3
  id+ : Inport  Port=4
  vq- : Inport  Port=5
  vd- : Inport  Port=6
  iq- : Inport  Port=7
  id- : Inport  Port=8
  Gain : Gain  Gain=3/2
  Gain1 : Gain  Gain=3/2
  Gain2 : Gain  Gain=-1
  Gain3 : Gain  Gain=-1
  Gain4 : Gain  Gain=negseq_en
  Mux{,1..3} (4 alike) : Mux  Inputs=2
  Product{,1..3} (4 alike) : Product
  Sum1 : Sum
  Sum2 : Sum
  Sum8 : Sum
  PQ : Outport
  wires:
  Sum8/1 -> Gain/1
  Gain2/1 -> Mux2/2
  Mux2/1 -> Product2/2
  Product2/1 -> Sum8/2
  Mux/1 -> Product/2
  Product/1 -> Sum8/1
  iq+/1 -> [iqp]
  [iqp] -> Gain2/1, Mux/1
  id+/1 -> [idp]
  [idp] -> Mux2/1, Mux/2
  vq+/1 -> [vqp]
  [vqp] -> Product/1
  vd+/1 -> [vdp]
  [vdp] -> Product2/1
  Gain/1 -> Sum1/1
  Sum1/1 -> PQ/1
  Gain3/1 -> Mux3/2
  Mux1/1 -> Product1/2
  Product3/1 -> Sum2/2
  Product1/1 -> Sum2/1
  [vdn] -> Product3/1
  Mux3/1 -> Product3/2
  [vqn] -> Product1/1
  Sum2/1 -> Gain1/1
  [iqn] -> Gain3/1, Mux1/1
  [idn] -> Mux3/1, Mux1/2
  vq-/1 -> [vqn]
  vd-/1 -> [vdn]
  iq-/1 -> [iqn]
  id-/1 -> [idn]
  Gain1/1 -> Gain4/1
  Gain4/1 -> Sum1/2

== system Scenario_3_v2/G7/VSC v2/VSC Control/Control loops/SW, EMT AVG, Phasor Quasi-EMT/Outer-loop/Power calculation ==
  note: AC power calculation using symmetrical components in dq axis
  note: Pavgp = 3/2*(vqp*iqp + vdp*idp) and Qavgp = 3/2*(vqp*idp-vdp*iqp)
  note: P = Pavg + Pc2*cos(2wt) + Ps2*sin(2wt) ---> Pavg = Pavgp + Pavgn
  note: Q = Qavg + Qc2*cos(2wt) + Qs2*sin(2wt) ---> Qavg = Qavgp + Qavgn
  note: Pavgn = 3/2*(vqn*iqn + vdn*idn) and Qavgn = 3/2*(vqn*idn-vdn*iqn)
  vq+ : Inport
  vd+ : Inport  Port=2
  iq+ : Inport  Port=3
  id+ : Inport  Port=4
  vq- : Inport  Port=5
  vd- : Inport  Port=6
  iq- : Inport  Port=7
  id- : Inport  Port=8
  Gain : Gain  Gain=3/2
  Gain1 : Gain  Gain=3/2
  Gain2 : Gain  Gain=-1
  Gain3 : Gain  Gain=-1
  Gain4 : Gain  Gain=negseq_en
  Mux{,1..3} (4 alike) : Mux  Inputs=2
  Product{,1..3} (4 alike) : Product
  Sum1 : Sum
  Sum2 : Sum
  Sum8 : Sum
  PQ : Outport
  wires:
  Sum8/1 -> Gain/1
  Gain2/1 -> Mux2/2
  Mux2/1 -> Product2/2
  Product2/1 -> Sum8/2
  Mux/1 -> Product/2
  Product/1 -> Sum8/1
  iq+/1 -> [iqp]
  [iqp] -> Gain2/1, Mux/1
  id+/1 -> [idp]
  [idp] -> Mux2/1, Mux/2
  vq+/1 -> [vqp]
  [vqp] -> Product/1
  vd+/1 -> [vdp]
  [vdp] -> Product2/1
  Gain/1 -> Sum1/1
  Sum1/1 -> PQ/1
  Gain3/1 -> Mux3/2
  Mux1/1 -> Product1/2
  Product3/1 -> Sum2/2
  Product1/1 -> Sum2/1
  [vdn] -> Product3/1
  Mux3/1 -> Product3/2
  [vqn] -> Product1/1
  Sum2/1 -> Gain1/1
  [iqn] -> Gain3/1, Mux1/1
  [idn] -> Mux3/1, Mux1/2
  vq-/1 -> [vqn]
  vd-/1 -> [vdn]
  iq-/1 -> [iqn]
  id-/1 -> [idn]
  Gain1/1 -> Gain4/1
  Gain4/1 -> Sum1/2

== system Scenario_3_v2/G7/VSC v2/VSC Control/Control loops/SW, EMT AVG, Phasor Quasi-EMT/Outer-loop/Subsystem2 ==
  note: Hold initial variable value for a given time
  In1 : Inport
  Constant : Constant  Value=x0
  Constant1 : Constant
  Integrator : Integrator
  Switch : Switch  Threshold=Td
  Out1 : Outport
  wires:
  Integrator/1 -> Switch/2
  In1/1 -> Switch/1
  Switch/1 -> Out1/1
  Constant/1 -> Switch/3
  Constant1/1 -> Integrator/1

== system Scenario_3_v2/G7/VSC v2/VSC Control/Control loops/SW, EMT AVG, Phasor Quasi-EMT/Outer-loop/Subsystem3 ==
  note: Hold initial variable value for a given time
  In1 : Inport
  Constant : Constant  Value=x0
  Constant1 : Constant
  Integrator : Integrator
  Switch : Switch  Threshold=Td
  Out1 : Outport
  wires:
  Integrator/1 -> Switch/2
  In1/1 -> Switch/1
  Switch/1 -> Out1/1
  Constant/1 -> Switch/3
  Constant1/1 -> Integrator/1

== system Scenario_3_v2/G7/VSC v2/VSC Control/Measurements/EMT/PLL aligned with positive-sequence/Phase-sequence separation ==
  note: Phase-sequence separation based on
      | Delayed Signal Cancellation (DSC) method
  abc : Inport
  Theta : Inport  Port=2
  Complex to Real-Imag1 : ComplexToRealImag
  Complex to Real-Imag2 : ComplexToRealImag
  Complex to Real-Imag3 : ComplexToRealImag
  Constant : Constant  Value=negseq_en
  Demux3 : Demux  Outputs=3
  Exp2 : Math  OutputSignalType=complex  SaturateOnIntegerOverflow=on
  Exp3 : Math  OutputSignalType=complex  SaturateOnIntegerOverflow=on
  Gain1 : Gain  Gain=1/2
  Gain4 : Gain  Gain=-1i
  Gain5 : Gain  Gain=1i
  Gain6 : Gain  Gain=1/2
  Gain7 : Gain  Gain=1i
  NOT : Logic  Operator=NOT  IconShape=distinctive  AllPortsSameDT=off  OutDataTypeStr=boolean
  Product3 : Product
  Product4 : Product
  Real-Imag to Complex : RealImagToComplex
  Real-Imag to Complex1 : RealImagToComplex
  Sum1 : Sum  Inputs=|++
  Sum2 : Sum  Inputs=-+|
  Switch : Switch  Criteria=u2 ~= 0
  Terminator3 : Terminator
  Transport Delay2 : TransportDelay  DelayTime=1/4*(1/fg)  BufferSize=1024*4
  Transport Delay3 : TransportDelay  DelayTime=1/4*(1/fg)  BufferSize=1024*4
  abc to Alpha-Beta-Zero : powerlib_meascontrol/Transformations/abc to Alpha-Beta-Zero
  q+ : Outport
  d+ : Outport  Port=2
  q- : Outport  Port=3
  d- : Outport  Port=4
  wires:
  NOT/1 -> Switch/2
  Constant/1 -> NOT/1
  Switch/1 -> Product3/1
  Gain6/1 -> Switch/3
  Sum2/1 -> Gain1/1
  Transport Delay2/1 -> Real-Imag to Complex1/1
  Demux3/1 -> Real-Imag to Complex/1
  Complex to Real-Imag1/2 -> Transport Delay3/1
  Gain1/1 -> Product4/2
  Real-Imag to Complex/1 -> Complex to Real-Imag1/1, Sum2/2, Sum1/1, Switch/1
  Complex to Real-Imag3/1 -> d-/1
  Real-Imag to Complex1/1 -> Gain5/1
  Complex to Real-Imag1/1 -> Transport Delay2/1
  Transport Delay3/1 -> Real-Imag to Complex1/2
  Demux3/2 -> Real-Imag to Complex/2
  Product3/1 -> Complex to Real-Imag2/1
  Product4/1 -> Complex to Real-Imag3/1
  abc to Alpha-Beta-Zero/1 -> Demux3/1
  abc/1 -> abc to Alpha-Beta-Zero/1
  Exp3/1 -> Product4/1
  Complex to Real-Imag3/2 -> q-/1
  Complex to Real-Imag2/2 -> q+/1
  Demux3/3 -> Terminator3/1
  Sum1/1 -> Gain6/1
  Gain5/1 -> Sum2/1, Sum1/2
  Exp2/1 -> Product3/2
  Gain4/1 -> Exp2/1
  Theta/1 -> Gain4/1, Gain7/1
  Gain7/1 -> Exp3/1
  Complex to Real-Imag2/1 -> d+/1

== system Scenario_3_v2/G7/VSC v2/VSC Control/Measurements/EMT/PLL aligned with positive-sequence/Subsystem ==
  note: PI controller with reset port and initial conditions restored after reset or after maximum/minimum values are reached
  in : Inport
  Reset : Inport  Port=2
  Compare To Constant2 : simulink/Logic and Bit Operations/Compare To Constant  relop=~=  const=0  OutDataTypeStr=boolean
  Constant2 : Constant  Value=2*pi*fg
  Gain : Gain  Gain=kp_pll
  Gain1 : Gain  Gain=kp_pll/tau_pll
  Integrator Limited : Integrator  ExternalReset=level  InitialCondition=2*pi*fg  UpperSaturationLimit=10.1*2*pi*fg  LowerSaturationLimit=0.09*2*pi*fg  ShowSaturationPort=on
  Memory1 : Memory
  NOT : Logic  Operator=NOT  IconShape=distinctive  AllPortsSameDT=off  OutDataTypeStr=boolean
  OR2 : Logic  Operator=OR  IconShape=distinctive  AllPortsSameDT=off  OutDataTypeStr=boolean
  Product : Product
  Sum : Sum
  Switch1 : Switch
  w : Outport
  wires:
  Switch1/1 -> w/1
  Product/1 -> Gain1/1, Gain/1
  Gain1/1 -> Integrator Limited/1
  Integrator Limited/2 -> Compare To Constant2/1, Switch1/2
  Compare To Constant2/1 -> Memory1/1
  OR2/1 -> Integrator Limited/2, NOT/1
  Constant2/1 -> Switch1/3
  Memory1/1 -> OR2/1
  Reset/1 -> OR2/2
  Gain/1 -> Sum/1
  Integrator Limited/1 -> Sum/2
  Sum/1 -> Switch1/1
  in/1 -> Product/1
  NOT/1 -> Product/2

== system Scenario_3_v2/G9/VSC v2/VSC Control/Control loops/Phasor I 1st/Outer-loop/Power calculation ==
  note: AC power calculation using symmetrical components in dq axis
  note: Pavgp = 3/2*(vqp*iqp + vdp*idp) and Qavgp = 3/2*(vqp*idp-vdp*iqp)
  note: P = Pavg + Pc2*cos(2wt) + Ps2*sin(2wt) ---> Pavg = Pavgp + Pavgn
  note: Q = Qavg + Qc2*cos(2wt) + Qs2*sin(2wt) ---> Qavg = Qavgp + Qavgn
  note: Pavgn = 3/2*(vqn*iqn + vdn*idn) and Qavgn = 3/2*(vqn*idn-vdn*iqn)
  vq+ : Inport
  vd+ : Inport  Port=2
  iq+ : Inport  Port=3
  id+ : Inport  Port=4
  vq- : Inport  Port=5
  vd- : Inport  Port=6
  iq- : Inport  Port=7
  id- : Inport  Port=8
  Gain : Gain  Gain=3/2
  Gain1 : Gain  Gain=3/2
  Gain2 : Gain  Gain=-1
  Gain3 : Gain  Gain=-1
  Gain4 : Gain  Gain=negseq_en
  Mux{,1..3} (4 alike) : Mux  Inputs=2
  Product{,1..3} (4 alike) : Product
  Sum1 : Sum
  Sum2 : Sum
  Sum8 : Sum
  PQ : Outport
  wires:
  Sum8/1 -> Gain/1
  Gain2/1 -> Mux2/2
  Mux2/1 -> Product2/2
  Product2/1 -> Sum8/2
  Mux/1 -> Product/2
  Product/1 -> Sum8/1
  iq+/1 -> [iqp]
  [iqp] -> Gain2/1, Mux/1
  id+/1 -> [idp]
  [idp] -> Mux2/1, Mux/2
  vq+/1 -> [vqp]
  [vqp] -> Product/1
  vd+/1 -> [vdp]
  [vdp] -> Product2/1
  Gain/1 -> Sum1/1
  Sum1/1 -> PQ/1
  Gain3/1 -> Mux3/2
  Mux1/1 -> Product1/2
  Product3/1 -> Sum2/2
  Product1/1 -> Sum2/1
  [vdn] -> Product3/1
  Mux3/1 -> Product3/2
  [vqn] -> Product1/1
  Sum2/1 -> Gain1/1
  [iqn] -> Gain3/1, Mux1/1
  [idn] -> Mux3/1, Mux1/2
  vq-/1 -> [vqn]
  vd-/1 -> [vdn]
  iq-/1 -> [iqn]
  id-/1 -> [idn]
  Gain1/1 -> Gain4/1
  Gain4/1 -> Sum1/2

== system Scenario_3_v2/G9/VSC v2/VSC Control/Control loops/Phasor I ref/Outer-loop/Power calculation ==
  note: AC power calculation using symmetrical components in dq axis
  note: Pavgp = 3/2*(vqp*iqp + vdp*idp) and Qavgp = 3/2*(vqp*idp-vdp*iqp)
  note: P = Pavg + Pc2*cos(2wt) + Ps2*sin(2wt) ---> Pavg = Pavgp + Pavgn
  note: Q = Qavg + Qc2*cos(2wt) + Qs2*sin(2wt) ---> Qavg = Qavgp + Qavgn
  note: Pavgn = 3/2*(vqn*iqn + vdn*idn) and Qavgn = 3/2*(vqn*idn-vdn*iqn)
  vq+ : Inport
  vd+ : Inport  Port=2
  iq+ : Inport  Port=3
  id+ : Inport  Port=4
  vq- : Inport  Port=5
  vd- : Inport  Port=6
  iq- : Inport  Port=7
  id- : Inport  Port=8
  Gain : Gain  Gain=3/2
  Gain1 : Gain  Gain=3/2
  Gain2 : Gain  Gain=-1
  Gain3 : Gain  Gain=-1
  Gain4 : Gain  Gain=negseq_en
  Mux{,1..3} (4 alike) : Mux  Inputs=2
  Product{,1..3} (4 alike) : Product
  Sum1 : Sum
  Sum2 : Sum
  Sum8 : Sum
  PQ : Outport
  wires:
  Sum8/1 -> Gain/1
  Gain2/1 -> Mux2/2
  Mux2/1 -> Product2/2
  Product2/1 -> Sum8/2
  Mux/1 -> Product/2
  Product/1 -> Sum8/1
  iq+/1 -> [iqp]
  [iqp] -> Gain2/1, Mux/1
  id+/1 -> [idp]
  [idp] -> Mux2/1, Mux/2
  vq+/1 -> [vqp]
  [vqp] -> Product/1
  vd+/1 -> [vdp]
  [vdp] -> Product2/1
  Gain/1 -> Sum1/1
  Sum1/1 -> PQ/1
  Gain3/1 -> Mux3/2
  Mux1/1 -> Product1/2
  Product3/1 -> Sum2/2
  Product1/1 -> Sum2/1
  [vdn] -> Product3/1
  Mux3/1 -> Product3/2
  [vqn] -> Product1/1
  Sum2/1 -> Gain1/1
  [iqn] -> Gain3/1, Mux1/1
  [idn] -> Mux3/1, Mux1/2
  vq-/1 -> [vqn]
  vd-/1 -> [vdn]
  iq-/1 -> [iqn]
  id-/1 -> [idn]
  Gain1/1 -> Gain4/1
  Gain4/1 -> Sum1/2

== system Scenario_3_v2/G9/VSC v2/VSC Control/Control loops/Phasor PQ 1st/Outer-loop/Power calculation ==
  note: AC power calculation using symmetrical components in dq axis
  note: Pavgp = 3/2*(vqp*iqp + vdp*idp) and Qavgp = 3/2*(vqp*idp-vdp*iqp)
  note: P = Pavg + Pc2*cos(2wt) + Ps2*sin(2wt) ---> Pavg = Pavgp + Pavgn
  note: Q = Qavg + Qc2*cos(2wt) + Qs2*sin(2wt) ---> Qavg = Qavgp + Qavgn
  note: Pavgn = 3/2*(vqn*iqn + vdn*idn) and Qavgn = 3/2*(vqn*idn-vdn*iqn)
  vq+ : Inport
  vd+ : Inport  Port=2
  iq+ : Inport  Port=3
  id+ : Inport  Port=4
  vq- : Inport  Port=5
  vd- : Inport  Port=6
  iq- : Inport  Port=7
  id- : Inport  Port=8
  Gain : Gain  Gain=3/2
  Gain1 : Gain  Gain=3/2
  Gain2 : Gain  Gain=-1
  Gain3 : Gain  Gain=-1
  Gain4 : Gain  Gain=negseq_en
  Mux{,1..3} (4 alike) : Mux  Inputs=2
  Product{,1..3} (4 alike) : Product
  Sum1 : Sum
  Sum2 : Sum
  Sum8 : Sum
  PQ : Outport
  wires:
  Sum8/1 -> Gain/1
  Gain2/1 -> Mux2/2
  Mux2/1 -> Product2/2
  Product2/1 -> Sum8/2
  Mux/1 -> Product/2
  Product/1 -> Sum8/1
  iq+/1 -> [iqp]
  [iqp] -> Gain2/1, Mux/1
  id+/1 -> [idp]
  [idp] -> Mux2/1, Mux/2
  vq+/1 -> [vqp]
  [vqp] -> Product/1
  vd+/1 -> [vdp]
  [vdp] -> Product2/1
  Gain/1 -> Sum1/1
  Sum1/1 -> PQ/1
  Gain3/1 -> Mux3/2
  Mux1/1 -> Product1/2
  Product3/1 -> Sum2/2
  Product1/1 -> Sum2/1
  [vdn] -> Product3/1
  Mux3/1 -> Product3/2
  [vqn] -> Product1/1
  Sum2/1 -> Gain1/1
  [iqn] -> Gain3/1, Mux1/1
  [idn] -> Mux3/1, Mux1/2
  vq-/1 -> [vqn]
  vd-/1 -> [vdn]
  iq-/1 -> [iqn]
  id-/1 -> [idn]
  Gain1/1 -> Gain4/1
  Gain4/1 -> Sum1/2

== system Scenario_3_v2/G9/VSC v2/VSC Control/Control loops/SW, EMT AVG, Phasor Quasi-EMT/Outer-loop/Power calculation ==
  note: AC power calculation using symmetrical components in dq axis
  note: Pavgp = 3/2*(vqp*iqp + vdp*idp) and Qavgp = 3/2*(vqp*idp-vdp*iqp)
  note: P = Pavg + Pc2*cos(2wt) + Ps2*sin(2wt) ---> Pavg = Pavgp + Pavgn
  note: Q = Qavg + Qc2*cos(2wt) + Qs2*sin(2wt) ---> Qavg = Qavgp + Qavgn
  note: Pavgn = 3/2*(vqn*iqn + vdn*idn) and Qavgn = 3/2*(vqn*idn-vdn*iqn)
  vq+ : Inport
  vd+ : Inport  Port=2
  iq+ : Inport  Port=3
  id+ : Inport  Port=4
  vq- : Inport  Port=5
  vd- : Inport  Port=6
  iq- : Inport  Port=7
  id- : Inport  Port=8
  Gain : Gain  Gain=3/2
  Gain1 : Gain  Gain=3/2
  Gain2 : Gain  Gain=-1
  Gain3 : Gain  Gain=-1
  Gain4 : Gain  Gain=negseq_en
  Mux{,1..3} (4 alike) : Mux  Inputs=2
  Product{,1..3} (4 alike) : Product
  Sum1 : Sum
  Sum2 : Sum
  Sum8 : Sum
  PQ : Outport
  wires:
  Sum8/1 -> Gain/1
  Gain2/1 -> Mux2/2
  Mux2/1 -> Product2/2
  Product2/1 -> Sum8/2
  Mux/1 -> Product/2
  Product/1 -> Sum8/1
  iq+/1 -> [iqp]
  [iqp] -> Gain2/1, Mux/1
  id+/1 -> [idp]
  [idp] -> Mux2/1, Mux/2
  vq+/1 -> [vqp]
  [vqp] -> Product/1
  vd+/1 -> [vdp]
  [vdp] -> Product2/1
  Gain/1 -> Sum1/1
  Sum1/1 -> PQ/1
  Gain3/1 -> Mux3/2
  Mux1/1 -> Product1/2
  Product3/1 -> Sum2/2
  Product1/1 -> Sum2/1
  [vdn] -> Product3/1
  Mux3/1 -> Product3/2
  [vqn] -> Product1/1
  Sum2/1 -> Gain1/1
  [iqn] -> Gain3/1, Mux1/1
  [idn] -> Mux3/1, Mux1/2
  vq-/1 -> [vqn]
  vd-/1 -> [vdn]
  iq-/1 -> [iqn]
  id-/1 -> [idn]
  Gain1/1 -> Gain4/1
  Gain4/1 -> Sum1/2

== system Scenario_3_v2/G9/VSC v2/VSC Control/Control loops/SW, EMT AVG, Phasor Quasi-EMT/Outer-loop/Subsystem2 ==
  note: Hold initial variable value for a given time
  In1 : Inport
  Constant : Constant  Value=x0
  Constant1 : Constant
  Integrator : Integrator
  Switch : Switch  Threshold=Td
  Out1 : Outport
  wires:
  Integrator/1 -> Switch/2
  In1/1 -> Switch/1
  Switch/1 -> Out1/1
  Constant/1 -> Switch/3
  Constant1/1 -> Integrator/1

== system Scenario_3_v2/G9/VSC v2/VSC Control/Control loops/SW, EMT AVG, Phasor Quasi-EMT/Outer-loop/Subsystem3 ==
  note: Hold initial variable value for a given time
  In1 : Inport
  Constant : Constant  Value=x0
  Constant1 : Constant
  Integrator : Integrator
  Switch : Switch  Threshold=Td
  Out1 : Outport
  wires:
  Integrator/1 -> Switch/2
  In1/1 -> Switch/1
  Switch/1 -> Out1/1
  Constant/1 -> Switch/3
  Constant1/1 -> Integrator/1

== system Scenario_3_v2/G9/VSC v2/VSC Control/Measurements/EMT/PLL aligned with positive-sequence/Phase-sequence separation ==
  note: Phase-sequence separation based on
      | Delayed Signal Cancellation (DSC) method
  abc : Inport
  Theta : Inport  Port=2
  Complex to Real-Imag1 : ComplexToRealImag
  Complex to Real-Imag2 : ComplexToRealImag
  Complex to Real-Imag3 : ComplexToRealImag
  Constant : Constant  Value=negseq_en
  Demux3 : Demux  Outputs=3
  Exp2 : Math  OutputSignalType=complex  SaturateOnIntegerOverflow=on
  Exp3 : Math  OutputSignalType=complex  SaturateOnIntegerOverflow=on
  Gain1 : Gain  Gain=1/2
  Gain4 : Gain  Gain=-1i
  Gain5 : Gain  Gain=1i
  Gain6 : Gain  Gain=1/2
  Gain7 : Gain  Gain=1i
  NOT : Logic  Operator=NOT  IconShape=distinctive  AllPortsSameDT=off  OutDataTypeStr=boolean
  Product3 : Product
  Product4 : Product
  Real-Imag to Complex : RealImagToComplex
  Real-Imag to Complex1 : RealImagToComplex
  Sum1 : Sum  Inputs=|++
  Sum2 : Sum  Inputs=-+|
  Switch : Switch  Criteria=u2 ~= 0
  Terminator3 : Terminator
  Transport Delay2 : TransportDelay  DelayTime=1/4*(1/fg)  BufferSize=1024*4
  Transport Delay3 : TransportDelay  DelayTime=1/4*(1/fg)  BufferSize=1024*4
  abc to Alpha-Beta-Zero : powerlib_meascontrol/Transformations/abc to Alpha-Beta-Zero
  q+ : Outport
  d+ : Outport  Port=2
  q- : Outport  Port=3
  d- : Outport  Port=4
  wires:
  NOT/1 -> Switch/2
  Constant/1 -> NOT/1
  Switch/1 -> Product3/1
  Gain6/1 -> Switch/3
  Sum2/1 -> Gain1/1
  Transport Delay2/1 -> Real-Imag to Complex1/1
  Demux3/1 -> Real-Imag to Complex/1
  Complex to Real-Imag1/2 -> Transport Delay3/1
  Gain1/1 -> Product4/2
  Real-Imag to Complex/1 -> Complex to Real-Imag1/1, Sum2/2, Sum1/1, Switch/1
  Complex to Real-Imag3/1 -> d-/1
  Real-Imag to Complex1/1 -> Gain5/1
  Complex to Real-Imag1/1 -> Transport Delay2/1
  Transport Delay3/1 -> Real-Imag to Complex1/2
  Demux3/2 -> Real-Imag to Complex/2
  Product3/1 -> Complex to Real-Imag2/1
  Product4/1 -> Complex to Real-Imag3/1
  abc to Alpha-Beta-Zero/1 -> Demux3/1
  abc/1 -> abc to Alpha-Beta-Zero/1
  Exp3/1 -> Product4/1
  Complex to Real-Imag3/2 -> q-/1
  Complex to Real-Imag2/2 -> q+/1
  Demux3/3 -> Terminator3/1
  Sum1/1 -> Gain6/1
  Gain5/1 -> Sum2/1, Sum1/2
  Exp2/1 -> Product3/2
  Gain4/1 -> Exp2/1
  Theta/1 -> Gain4/1, Gain7/1
  Gain7/1 -> Exp3/1
  Complex to Real-Imag2/1 -> d+/1

== system Scenario_3_v2/G9/VSC v2/VSC Control/Measurements/EMT/PLL aligned with positive-sequence/Subsystem ==
  note: PI controller with reset port and initial conditions restored after reset or after maximum/minimum values are reached
  in : Inport
  Reset : Inport  Port=2
  Compare To Constant2 : simulink/Logic and Bit Operations/Compare To Constant  relop=~=  const=0  OutDataTypeStr=boolean
  Constant2 : Constant  Value=2*pi*fg
  Gain : Gain  Gain=kp_pll
  Gain1 : Gain  Gain=kp_pll/tau_pll
  Integrator Limited : Integrator  ExternalReset=level  InitialCondition=2*pi*fg  UpperSaturationLimit=10.1*2*pi*fg  LowerSaturationLimit=0.09*2*pi*fg  ShowSaturationPort=on
  Memory1 : Memory
  NOT : Logic  Operator=NOT  IconShape=distinctive  AllPortsSameDT=off  OutDataTypeStr=boolean
  OR2 : Logic  Operator=OR  IconShape=distinctive  AllPortsSameDT=off  OutDataTypeStr=boolean
  Product : Product
  Sum : Sum
  Switch1 : Switch
  w : Outport
  wires:
  Switch1/1 -> w/1
  Product/1 -> Gain1/1, Gain/1
  Gain1/1 -> Integrator Limited/1
  Integrator Limited/2 -> Compare To Constant2/1, Switch1/2
  Compare To Constant2/1 -> Memory1/1
  OR2/1 -> Integrator Limited/2, NOT/1
  Constant2/1 -> Switch1/3
  Memory1/1 -> OR2/1
  Reset/1 -> OR2/2
  Gain/1 -> Sum/1
  Integrator Limited/1 -> Sum/2
  Sum/1 -> Switch1/1
  in/1 -> Product/1
  NOT/1 -> Product/2
